simulink model "qpsk"  (R2021a)
settings: Solver=FixedStepDiscrete  StartTime=0.0  StopTime=1e-3  FixedStep=1/sampling_freq  RelTol=1e-3
undefined symbols (not defined in the file): coeff, data_rate, nco_21, sample_ratio, sampling_freq
libraries: simulink x6, simulink_extras x5, dspswit3 x2, commchan3 x1, commrandsrc2 x1, commsink2 x1
settings Model: SimulationMode=accelerator  Creator=Administrator  LastModifiedBy=Administrator

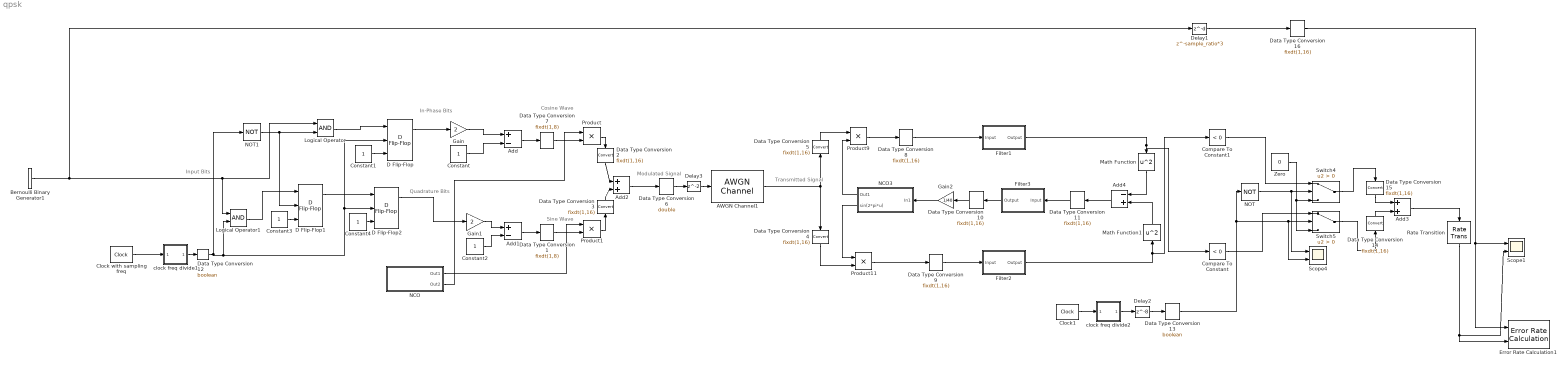
== system qpsk ==
  note: Transmitted Signal
  note: Quadrature Bits
  note: In-Phase Bits
  note: Input Bits
  note: Modulated Signal
  note: Cosine Wave
  note: Sine Wave
  AWGN Channel1 : commchan3/AWGN Channel  InputProcessing=Columns as channels (frame based)  seed=532  noiseMode="Signal to noise ratio  (Eb/No)"  EbNodB=SNR  EsNodB=10  SNRdB=SNR  bitsPerSym=1  Ps=1  Tsym=1/data_rate  variance=1
  Add : Sum  Inputs=+-
  Add1 : Sum  Inputs=+-
  Add2 : Sum
  Add3 : Sum
  Add4 : Sum  Inputs=-+
  Bernoulli Binary Generator1 : commrandsrc2/Bernoulli Binary Generator  P=0.3  seed=14  Ts=1/data_rate  frameBased=off  sampPerFrame=1  orient=off  outDataType=boolean
      settings: SourceProductBaseCode=CM
  Clock with sampling freq : simulink_extras/Flip Flops/Clock  period=1/sampling_freq*2
  Clock1 : simulink_extras/Flip Flops/Clock  period=1/sampling_freq*2
  Compare To Constant : simulink/Logic and Bit Operations/Compare To Constant  relop=<  const=0  OutDataTypeStr=boolean
  Compare To Constant1 : simulink/Logic and Bit Operations/Compare To Constant  relop=<  const=0  OutDataTypeStr=boolean
  Constant : Constant
  Constant1 : Constant  OutDataTypeStr=boolean
  Constant2 : Constant
  Constant3 : Constant  OutDataTypeStr=boolean
  Constant4 : Constant  OutDataTypeStr=boolean
  D Flip-Flop : simulink_extras/Flip Flops/D Flip-Flop
  D Flip-Flop1 : simulink_extras/Flip Flops/D Flip-Flop
  D Flip-Flop2 : simulink_extras/Flip Flops/D Flip-Flop
  Data Type Conversion1 : DataTypeConversion  OutMax=[1]  OutDataTypeStr=fixdt(1,8)
  Data Type Conversion{2..5,8..11,14..16} (11 alike) : DataTypeConversion  OutMax=[1]  OutDataTypeStr=fixdt(1,16)
  Data Type Conversion12 : DataTypeConversion  OutMax=[1]  OutDataTypeStr=boolean
  Data Type Conversion13 : DataTypeConversion  OutMax=[1]  OutDataTypeStr=boolean
  Data Type Conversion6 : DataTypeConversion  OutDataTypeStr=double  LockScale=on
  Data Type Conversion7 : DataTypeConversion  OutMax=[1]  OutDataTypeStr=fixdt(1,8)
  Delay1 : Delay  DelayLength=sample_ratio*3  SampleTime=1/sampling_freq
  Delay2 : Delay  DelayLength=8  SampleTime=1/sampling_freq
  Delay3 : Delay  SampleTime=1/sampling_freq
  Error Rate Calculation1 : commsink2/Error Rate Calculation  N=0  st_delay=20000  cp_mode=Entire frame  subframe=[]  PMode=Workspace  WsName=ErrorVec_QPSK  RsMode2=off  stop=off  numErr=100  maxBits=1e6
  Filter1 : Subsystem  Tag=FilterWizardSubSystem
      settings: ErrorFcn=dspFilterRealizedInBasicElemsAlgLoopErrFcnCallback
  Filter2 : Subsystem  Tag=FilterWizardSubSystem
      settings: ErrorFcn=dspFilterRealizedInBasicElemsAlgLoopErrFcnCallback
  Filter3 : Subsystem  Tag=FilterWizardSubSystem
      settings: ErrorFcn=dspFilterRealizedInBasicElemsAlgLoopErrFcnCallback
  Gain : Gain  Gain=2
  Gain1 : Gain  Gain=2
  Gain2 : Gain  Gain=1/40
  Logical Operator : Logic  AllPortsSameDT=off  OutDataTypeStr=boolean
  Logical Operator1 : Logic  AllPortsSameDT=off  OutDataTypeStr=boolean
  Math Function : Math  Operator=square  SignedPower=on  SaturateOnIntegerOverflow=on
  Math Function1 : Math  Operator=square  SignedPower=on  SaturateOnIntegerOverflow=on
  NCO : Subsystem
  NCO3 : Subsystem
  NOT : Logic  Operator=NOT  IconShape=distinctive  AllPortsSameDT=off  OutDataTypeStr=boolean
  NOT1 : Logic  Operator=NOT  IconShape=distinctive  AllPortsSameDT=off  OutDataTypeStr=boolean
  Product{,1,9,11} (4 alike) : Product
  Rate Transition : RateTransition  OutPortSampleTime=1/data_rate
  Scope1 : Scope  NumInputPorts=2
  Scope4 : Scope  NumInputPorts=2
  Switch4 : Switch  Criteria=u2 > Threshold
  Switch5 : Switch  Criteria=u2 > Threshold
  Zero : Constant  Value=0  OutDataTypeStr=fixdt(1,16,12)
  clock freq divide1 : Subsystem
  clock freq divide2 : Subsystem
  wires:
  Constant/1 -> Add/2
  Gain/1 -> Add/1
  Gain1/1 -> Add1/1
  Constant2/1 -> Add1/2
  Add/1 -> Data Type Conversion7/1
  Add1/1 -> Data Type Conversion1/1
  Product/1 -> Data Type Conversion2/1
  Product1/1 -> Data Type Conversion3/1
  Add2/1 -> Data Type Conversion6/1
  Product9/1 -> Data Type Conversion8/1
  Product11/1 -> Data Type Conversion9/1
  AWGN Channel1/1 -> Data Type Conversion4/1, Data Type Conversion5/1
  Data Type Conversion7/1 -> Product/2
  Data Type Conversion1/1 -> Product1/2
  Data Type Conversion2/1 -> Add2/1
  Data Type Conversion3/1 -> Add2/2
  Data Type Conversion4/1 -> Product11/2
  Data Type Conversion5/1 -> Product9/1
  Data Type Conversion6/1 -> Delay3/1
  NCO3/1(Out1) -> Product9/2
  NCO3/2(sin(2*pi*u)) -> Product11/1
  NCO/2(Out2) -> Product/1
  Data Type Conversion8/1 -> Filter1/1(Input)
  Data Type Conversion9/1 -> Filter2/1(Input)
  Gain2/1 -> NCO3/1(In1)
  Data Type Conversion11/1 -> Filter3/1(Input)
  Constant4/1 -> D Flip-Flop2/3
  D Flip-Flop/1 -> Gain/1
  Constant1/1 -> D Flip-Flop/3
  Constant3/1 -> D Flip-Flop1/3
  Logical Operator/1 -> D Flip-Flop/1
  NOT1/1 -> D Flip-Flop1/2, Logical Operator/2
  Logical Operator1/1 -> D Flip-Flop1/1
  D Flip-Flop2/1 -> Gain1/1
  D Flip-Flop1/1 -> D Flip-Flop2/1
  Clock with sampling freq/1 -> clock freq divide1/1(In1)
  Data Type Conversion12/1 -> NOT1/1, D Flip-Flop/2, D Flip-Flop2/2, Logical Operator1/2
  Delay1/1 -> Data Type Conversion16/1
  Delay2/1 -> Data Type Conversion13/1
  Compare To Constant1/1 -> Switch4/1
  Data Type Conversion14/1 -> Add3/2
  Data Type Conversion15/1 -> Add3/1
  Data Type Conversion16/1 -> Error Rate Calculation1/1, Scope1/1
  Add3/1 -> Rate Transition/1
  NCO/1(Out1) -> Product1/1
  Math Function/1 -> Add4/1
  Math Function1/1 -> Add4/2
  Add4/1 -> Data Type Conversion11/1
  Data Type Conversion13/1 -> NOT/1, Scope4/2, Switch5/2
  NOT/1 -> Scope4/1, Switch4/2
  Compare To Constant/1 -> Switch5/1
  Zero/1 -> Switch5/3, Switch4/3
  Switch4/1 -> Data Type Conversion15/1
  Switch5/1 -> Data Type Conversion14/1
  Delay3/1 -> AWGN Channel1/1
  Filter1/1(Output) -> Compare To Constant/1, Math Function/1
  Filter2/1(Output) -> Compare To Constant1/1, Math Function1/1
  Filter3/1(Output) -> Data Type Conversion10/1
  Data Type Conversion10/1 -> Gain2/1
  Bernoulli Binary Generator1/1 -> Logical Operator/1, Logical Operator1/1, Delay1/1
  Rate Transition/1 -> Scope1/2, Error Rate Calculation1/2
  clock freq divide1/1(Out1) -> Data Type Conversion12/1
  Clock1/1 -> clock freq divide2/1(In1)
  clock freq divide2/1(Out1) -> Delay2/1

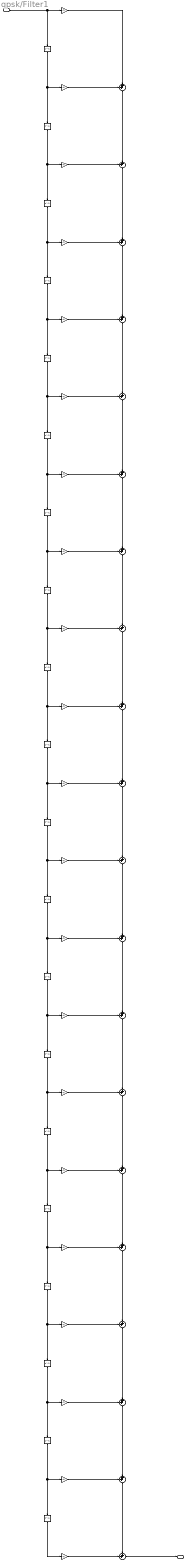
== system qpsk/Filter1 ==
  Input : Inport
  BodyDelay{2..21} (20 alike) : Delay  DelayLength=1  InitialCondition=0  InputProcessing=Columns as channels (frame based)  SampleTime=1/sampling_freq
  BodyLSum{2..21} (20 alike) : Sum  Inputs=++|  RndMeth=Nearest  SaturateOnIntegerOverflow=on  OutDataTypeStr=Inherit: Same as first input
  b(1) : Gain  Gain=coeff(1)  ParamDataTypeStr=double  RndMeth=Nearest  SaturateOnIntegerOverflow=on  OutDataTypeStr=Inherit: Same as input
  b(10) : Gain  Gain=coeff(10)  ParamDataTypeStr=double  RndMeth=Nearest  SaturateOnIntegerOverflow=on  OutDataTypeStr=Inherit: Same as input
  b(11) : Gain  Gain=coeff(11)  ParamDataTypeStr=double  RndMeth=Nearest  SaturateOnIntegerOverflow=on  OutDataTypeStr=Inherit: Same as input
  b(12) : Gain  Gain=coeff(12)  ParamDataTypeStr=double  RndMeth=Nearest  SaturateOnIntegerOverflow=on  OutDataTypeStr=Inherit: Same as input
  b(13) : Gain  Gain=coeff(13)  ParamDataTypeStr=double  RndMeth=Nearest  SaturateOnIntegerOverflow=on  OutDataTypeStr=Inherit: Same as input
  b(14) : Gain  Gain=coeff(14)  ParamDataTypeStr=double  RndMeth=Nearest  SaturateOnIntegerOverflow=on  OutDataTypeStr=Inherit: Same as input
  b(15) : Gain  Gain=coeff(15)  ParamDataTypeStr=double  RndMeth=Nearest  SaturateOnIntegerOverflow=on  OutDataTypeStr=Inherit: Same as input
  b(16) : Gain  Gain=coeff(16)  ParamDataTypeStr=double  RndMeth=Nearest  SaturateOnIntegerOverflow=on  OutDataTypeStr=Inherit: Same as input
  b(17) : Gain  Gain=coeff(17)  ParamDataTypeStr=double  RndMeth=Nearest  SaturateOnIntegerOverflow=on  OutDataTypeStr=Inherit: Same as input
  b(18) : Gain  Gain=coeff(18)  ParamDataTypeStr=double  RndMeth=Nearest  SaturateOnIntegerOverflow=on  OutDataTypeStr=Inherit: Same as input
  b(19) : Gain  Gain=coeff(19)  ParamDataTypeStr=double  RndMeth=Nearest  SaturateOnIntegerOverflow=on  OutDataTypeStr=Inherit: Same as input
  b(2) : Gain  Gain=coeff(2)  ParamDataTypeStr=double  RndMeth=Nearest  SaturateOnIntegerOverflow=on  OutDataTypeStr=Inherit: Same as input
  b(20) : Gain  Gain=coeff(20)  ParamDataTypeStr=double  RndMeth=Nearest  SaturateOnIntegerOverflow=on  OutDataTypeStr=Inherit: Same as input
  b(21) : Gain  Gain=coeff(21)  ParamDataTypeStr=double  RndMeth=Nearest  SaturateOnIntegerOverflow=on  OutDataTypeStr=Inherit: Same as input
  b(3) : Gain  Gain=coeff(3)  ParamDataTypeStr=double  RndMeth=Nearest  SaturateOnIntegerOverflow=on  OutDataTypeStr=Inherit: Same as input
  b(4) : Gain  Gain=coeff(4)  ParamDataTypeStr=double  RndMeth=Nearest  SaturateOnIntegerOverflow=on  OutDataTypeStr=Inherit: Same as input
  b(5) : Gain  Gain=coeff(5)  ParamDataTypeStr=double  RndMeth=Nearest  SaturateOnIntegerOverflow=on  OutDataTypeStr=Inherit: Same as input
  b(6) : Gain  Gain=coeff(6)  ParamDataTypeStr=double  RndMeth=Nearest  SaturateOnIntegerOverflow=on  OutDataTypeStr=Inherit: Same as input
  b(7) : Gain  Gain=coeff(7)  ParamDataTypeStr=double  RndMeth=Nearest  SaturateOnIntegerOverflow=on  OutDataTypeStr=Inherit: Same as input
  b(8) : Gain  Gain=coeff(8)  ParamDataTypeStr=double  RndMeth=Nearest  SaturateOnIntegerOverflow=on  OutDataTypeStr=Inherit: Same as input
  b(9) : Gain  Gain=coeff(9)  ParamDataTypeStr=double  RndMeth=Nearest  SaturateOnIntegerOverflow=on  OutDataTypeStr=Inherit: Same as input
  Output : Outport
  wires:
  Input/1 -> b(1)/1, BodyDelay2/1
  b(1)/1 -> BodyLSum2/2
  BodyDelay2/1 -> b(2)/1, BodyDelay3/1
  b(2)/1 -> BodyLSum2/1
  BodyLSum2/1 -> BodyLSum3/2
  BodyDelay3/1 -> b(3)/1, BodyDelay4/1
  b(3)/1 -> BodyLSum3/1
  BodyLSum3/1 -> BodyLSum4/2
  BodyDelay4/1 -> b(4)/1, BodyDelay5/1
  b(4)/1 -> BodyLSum4/1
  BodyLSum4/1 -> BodyLSum5/2
  BodyDelay5/1 -> b(5)/1, BodyDelay6/1
  b(5)/1 -> BodyLSum5/1
  BodyLSum5/1 -> BodyLSum6/2
  BodyDelay6/1 -> b(6)/1, BodyDelay7/1
  b(6)/1 -> BodyLSum6/1
  BodyLSum6/1 -> BodyLSum7/2
  BodyDelay7/1 -> b(7)/1, BodyDelay8/1
  b(7)/1 -> BodyLSum7/1
  BodyLSum7/1 -> BodyLSum8/2
  BodyDelay8/1 -> b(8)/1, BodyDelay9/1
  b(8)/1 -> BodyLSum8/1
  BodyLSum8/1 -> BodyLSum9/2
  BodyDelay9/1 -> b(9)/1, BodyDelay10/1
  b(9)/1 -> BodyLSum9/1
  BodyLSum9/1 -> BodyLSum10/2
  BodyDelay10/1 -> b(10)/1, BodyDelay11/1
  b(10)/1 -> BodyLSum10/1
  BodyLSum10/1 -> BodyLSum11/2
  BodyDelay11/1 -> b(11)/1, BodyDelay12/1
  b(11)/1 -> BodyLSum11/1
  BodyLSum11/1 -> BodyLSum12/2
  BodyDelay12/1 -> b(12)/1, BodyDelay13/1
  b(12)/1 -> BodyLSum12/1
  BodyLSum12/1 -> BodyLSum13/2
  BodyDelay13/1 -> b(13)/1, BodyDelay14/1
  b(13)/1 -> BodyLSum13/1
  BodyLSum13/1 -> BodyLSum14/2
  BodyDelay14/1 -> b(14)/1, BodyDelay15/1
  b(14)/1 -> BodyLSum14/1
  BodyLSum14/1 -> BodyLSum15/2
  BodyDelay15/1 -> b(15)/1, BodyDelay16/1
  b(15)/1 -> BodyLSum15/1
  BodyLSum15/1 -> BodyLSum16/2
  BodyDelay16/1 -> b(16)/1, BodyDelay17/1
  b(16)/1 -> BodyLSum16/1
  BodyLSum16/1 -> BodyLSum17/2
  BodyDelay17/1 -> b(17)/1, BodyDelay18/1
  b(17)/1 -> BodyLSum17/1
  BodyLSum17/1 -> BodyLSum18/2
  BodyDelay18/1 -> b(18)/1, BodyDelay19/1
  b(18)/1 -> BodyLSum18/1
  BodyLSum18/1 -> BodyLSum19/2
  BodyDelay19/1 -> b(19)/1, BodyDelay20/1
  b(19)/1 -> BodyLSum19/1
  BodyLSum19/1 -> BodyLSum20/2
  BodyDelay20/1 -> b(20)/1, BodyDelay21/1
  b(20)/1 -> BodyLSum20/1
  BodyLSum20/1 -> BodyLSum21/1
  BodyDelay21/1 -> b(21)/1
  b(21)/1 -> BodyLSum21/2
  BodyLSum21/1 -> Output/1

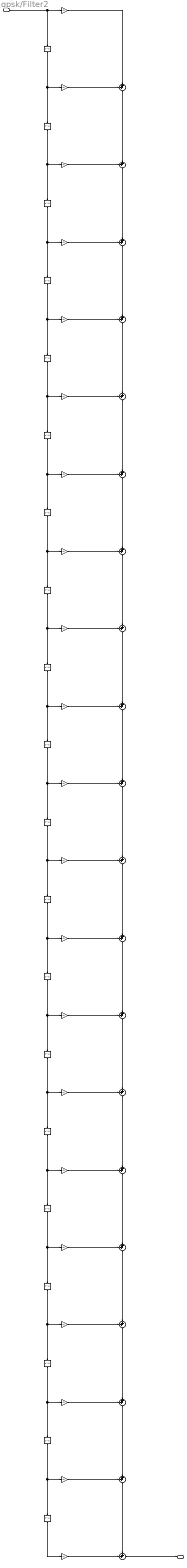
== system qpsk/Filter2 ==
  Input : Inport
  BodyDelay{2..21} (20 alike) : Delay  DelayLength=1  InitialCondition=0  InputProcessing=Columns as channels (frame based)  SampleTime=1/sampling_freq
  BodyLSum{2..21} (20 alike) : Sum  Inputs=++|  RndMeth=Nearest  SaturateOnIntegerOverflow=on  OutDataTypeStr=Inherit: Same as first input
  b(1) : Gain  Gain=coeff(1)  ParamDataTypeStr=double  RndMeth=Nearest  SaturateOnIntegerOverflow=on  OutDataTypeStr=Inherit: Same as input
  b(10) : Gain  Gain=coeff(10)  ParamDataTypeStr=double  RndMeth=Nearest  SaturateOnIntegerOverflow=on  OutDataTypeStr=Inherit: Same as input
  b(11) : Gain  Gain=coeff(11)  ParamDataTypeStr=double  RndMeth=Nearest  SaturateOnIntegerOverflow=on  OutDataTypeStr=Inherit: Same as input
  b(12) : Gain  Gain=coeff(12)  ParamDataTypeStr=double  RndMeth=Nearest  SaturateOnIntegerOverflow=on  OutDataTypeStr=Inherit: Same as input
  b(13) : Gain  Gain=coeff(13)  ParamDataTypeStr=double  RndMeth=Nearest  SaturateOnIntegerOverflow=on  OutDataTypeStr=Inherit: Same as input
  b(14) : Gain  Gain=coeff(14)  ParamDataTypeStr=double  RndMeth=Nearest  SaturateOnIntegerOverflow=on  OutDataTypeStr=Inherit: Same as input
  b(15) : Gain  Gain=coeff(15)  ParamDataTypeStr=double  RndMeth=Nearest  SaturateOnIntegerOverflow=on  OutDataTypeStr=Inherit: Same as input
  b(16) : Gain  Gain=coeff(16)  ParamDataTypeStr=double  RndMeth=Nearest  SaturateOnIntegerOverflow=on  OutDataTypeStr=Inherit: Same as input
  b(17) : Gain  Gain=coeff(17)  ParamDataTypeStr=double  RndMeth=Nearest  SaturateOnIntegerOverflow=on  OutDataTypeStr=Inherit: Same as input
  b(18) : Gain  Gain=coeff(18)  ParamDataTypeStr=double  RndMeth=Nearest  SaturateOnIntegerOverflow=on  OutDataTypeStr=Inherit: Same as input
  b(19) : Gain  Gain=coeff(19)  ParamDataTypeStr=double  RndMeth=Nearest  SaturateOnIntegerOverflow=on  OutDataTypeStr=Inherit: Same as input
  b(2) : Gain  Gain=coeff(2)  ParamDataTypeStr=double  RndMeth=Nearest  SaturateOnIntegerOverflow=on  OutDataTypeStr=Inherit: Same as input
  b(20) : Gain  Gain=coeff(20)  ParamDataTypeStr=double  RndMeth=Nearest  SaturateOnIntegerOverflow=on  OutDataTypeStr=Inherit: Same as input
  b(21) : Gain  Gain=coeff(21)  ParamDataTypeStr=double  RndMeth=Nearest  SaturateOnIntegerOverflow=on  OutDataTypeStr=Inherit: Same as input
  b(3) : Gain  Gain=coeff(3)  ParamDataTypeStr=double  RndMeth=Nearest  SaturateOnIntegerOverflow=on  OutDataTypeStr=Inherit: Same as input
  b(4) : Gain  Gain=coeff(4)  ParamDataTypeStr=double  RndMeth=Nearest  SaturateOnIntegerOverflow=on  OutDataTypeStr=Inherit: Same as input
  b(5) : Gain  Gain=coeff(5)  ParamDataTypeStr=double  RndMeth=Nearest  SaturateOnIntegerOverflow=on  OutDataTypeStr=Inherit: Same as input
  b(6) : Gain  Gain=coeff(6)  ParamDataTypeStr=double  RndMeth=Nearest  SaturateOnIntegerOverflow=on  OutDataTypeStr=Inherit: Same as input
  b(7) : Gain  Gain=coeff(7)  ParamDataTypeStr=double  RndMeth=Nearest  SaturateOnIntegerOverflow=on  OutDataTypeStr=Inherit: Same as input
  b(8) : Gain  Gain=coeff(8)  ParamDataTypeStr=double  RndMeth=Nearest  SaturateOnIntegerOverflow=on  OutDataTypeStr=Inherit: Same as input
  b(9) : Gain  Gain=coeff(9)  ParamDataTypeStr=double  RndMeth=Nearest  SaturateOnIntegerOverflow=on  OutDataTypeStr=Inherit: Same as input
  Output : Outport
  wires:
  Input/1 -> b(1)/1, BodyDelay2/1
  b(1)/1 -> BodyLSum2/2
  BodyDelay2/1 -> b(2)/1, BodyDelay3/1
  b(2)/1 -> BodyLSum2/1
  BodyLSum2/1 -> BodyLSum3/2
  BodyDelay3/1 -> b(3)/1, BodyDelay4/1
  b(3)/1 -> BodyLSum3/1
  BodyLSum3/1 -> BodyLSum4/2
  BodyDelay4/1 -> b(4)/1, BodyDelay5/1
  b(4)/1 -> BodyLSum4/1
  BodyLSum4/1 -> BodyLSum5/2
  BodyDelay5/1 -> b(5)/1, BodyDelay6/1
  b(5)/1 -> BodyLSum5/1
  BodyLSum5/1 -> BodyLSum6/2
  BodyDelay6/1 -> b(6)/1, BodyDelay7/1
  b(6)/1 -> BodyLSum6/1
  BodyLSum6/1 -> BodyLSum7/2
  BodyDelay7/1 -> b(7)/1, BodyDelay8/1
  b(7)/1 -> BodyLSum7/1
  BodyLSum7/1 -> BodyLSum8/2
  BodyDelay8/1 -> b(8)/1, BodyDelay9/1
  b(8)/1 -> BodyLSum8/1
  BodyLSum8/1 -> BodyLSum9/2
  BodyDelay9/1 -> b(9)/1, BodyDelay10/1
  b(9)/1 -> BodyLSum9/1
  BodyLSum9/1 -> BodyLSum10/2
  BodyDelay10/1 -> b(10)/1, BodyDelay11/1
  b(10)/1 -> BodyLSum10/1
  BodyLSum10/1 -> BodyLSum11/2
  BodyDelay11/1 -> b(11)/1, BodyDelay12/1
  b(11)/1 -> BodyLSum11/1
  BodyLSum11/1 -> BodyLSum12/2
  BodyDelay12/1 -> b(12)/1, BodyDelay13/1
  b(12)/1 -> BodyLSum12/1
  BodyLSum12/1 -> BodyLSum13/2
  BodyDelay13/1 -> b(13)/1, BodyDelay14/1
  b(13)/1 -> BodyLSum13/1
  BodyLSum13/1 -> BodyLSum14/2
  BodyDelay14/1 -> b(14)/1, BodyDelay15/1
  b(14)/1 -> BodyLSum14/1
  BodyLSum14/1 -> BodyLSum15/2
  BodyDelay15/1 -> b(15)/1, BodyDelay16/1
  b(15)/1 -> BodyLSum15/1
  BodyLSum15/1 -> BodyLSum16/2
  BodyDelay16/1 -> b(16)/1, BodyDelay17/1
  b(16)/1 -> BodyLSum16/1
  BodyLSum16/1 -> BodyLSum17/2
  BodyDelay17/1 -> b(17)/1, BodyDelay18/1
  b(17)/1 -> BodyLSum17/1
  BodyLSum17/1 -> BodyLSum18/2
  BodyDelay18/1 -> b(18)/1, BodyDelay19/1
  b(18)/1 -> BodyLSum18/1
  BodyLSum18/1 -> BodyLSum19/2
  BodyDelay19/1 -> b(19)/1, BodyDelay20/1
  b(19)/1 -> BodyLSum19/1
  BodyLSum19/1 -> BodyLSum20/2
  BodyDelay20/1 -> b(20)/1, BodyDelay21/1
  b(20)/1 -> BodyLSum20/1
  BodyLSum20/1 -> BodyLSum21/1
  BodyDelay21/1 -> b(21)/1
  b(21)/1 -> BodyLSum21/2
  BodyLSum21/1 -> Output/1

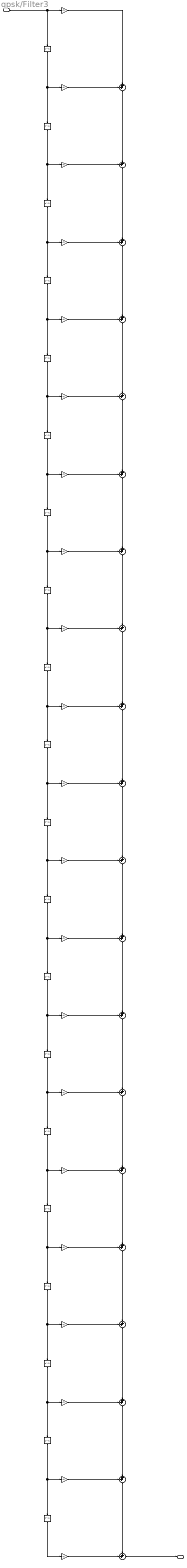
== system qpsk/Filter3 ==
  Input : Inport
  BodyDelay{2..21} (20 alike) : Delay  DelayLength=1  InitialCondition=0  InputProcessing=Columns as channels (frame based)  SampleTime=1/sampling_freq
  BodyLSum{2..21} (20 alike) : Sum  Inputs=++|  RndMeth=Nearest  SaturateOnIntegerOverflow=on  OutDataTypeStr=Inherit: Same as first input
  b(1) : Gain  Gain=coeff(1)  ParamDataTypeStr=double  RndMeth=Nearest  SaturateOnIntegerOverflow=on  OutDataTypeStr=Inherit: Same as input
  b(10) : Gain  Gain=coeff(10)  ParamDataTypeStr=double  RndMeth=Nearest  SaturateOnIntegerOverflow=on  OutDataTypeStr=Inherit: Same as input
  b(11) : Gain  Gain=coeff(11)  ParamDataTypeStr=double  RndMeth=Nearest  SaturateOnIntegerOverflow=on  OutDataTypeStr=Inherit: Same as input
  b(12) : Gain  Gain=coeff(12)  ParamDataTypeStr=double  RndMeth=Nearest  SaturateOnIntegerOverflow=on  OutDataTypeStr=Inherit: Same as input
  b(13) : Gain  Gain=coeff(13)  ParamDataTypeStr=double  RndMeth=Nearest  SaturateOnIntegerOverflow=on  OutDataTypeStr=Inherit: Same as input
  b(14) : Gain  Gain=coeff(14)  ParamDataTypeStr=double  RndMeth=Nearest  SaturateOnIntegerOverflow=on  OutDataTypeStr=Inherit: Same as input
  b(15) : Gain  Gain=coeff(15)  ParamDataTypeStr=double  RndMeth=Nearest  SaturateOnIntegerOverflow=on  OutDataTypeStr=Inherit: Same as input
  b(16) : Gain  Gain=coeff(16)  ParamDataTypeStr=double  RndMeth=Nearest  SaturateOnIntegerOverflow=on  OutDataTypeStr=Inherit: Same as input
  b(17) : Gain  Gain=coeff(17)  ParamDataTypeStr=double  RndMeth=Nearest  SaturateOnIntegerOverflow=on  OutDataTypeStr=Inherit: Same as input
  b(18) : Gain  Gain=coeff(18)  ParamDataTypeStr=double  RndMeth=Nearest  SaturateOnIntegerOverflow=on  OutDataTypeStr=Inherit: Same as input
  b(19) : Gain  Gain=coeff(19)  ParamDataTypeStr=double  RndMeth=Nearest  SaturateOnIntegerOverflow=on  OutDataTypeStr=Inherit: Same as input
  b(2) : Gain  Gain=coeff(2)  ParamDataTypeStr=double  RndMeth=Nearest  SaturateOnIntegerOverflow=on  OutDataTypeStr=Inherit: Same as input
  b(20) : Gain  Gain=coeff(20)  ParamDataTypeStr=double  RndMeth=Nearest  SaturateOnIntegerOverflow=on  OutDataTypeStr=Inherit: Same as input
  b(21) : Gain  Gain=coeff(21)  ParamDataTypeStr=double  RndMeth=Nearest  SaturateOnIntegerOverflow=on  OutDataTypeStr=Inherit: Same as input
  b(3) : Gain  Gain=coeff(3)  ParamDataTypeStr=double  RndMeth=Nearest  SaturateOnIntegerOverflow=on  OutDataTypeStr=Inherit: Same as input
  b(4) : Gain  Gain=coeff(4)  ParamDataTypeStr=double  RndMeth=Nearest  SaturateOnIntegerOverflow=on  OutDataTypeStr=Inherit: Same as input
  b(5) : Gain  Gain=coeff(5)  ParamDataTypeStr=double  RndMeth=Nearest  SaturateOnIntegerOverflow=on  OutDataTypeStr=Inherit: Same as input
  b(6) : Gain  Gain=coeff(6)  ParamDataTypeStr=double  RndMeth=Nearest  SaturateOnIntegerOverflow=on  OutDataTypeStr=Inherit: Same as input
  b(7) : Gain  Gain=coeff(7)  ParamDataTypeStr=double  RndMeth=Nearest  SaturateOnIntegerOverflow=on  OutDataTypeStr=Inherit: Same as input
  b(8) : Gain  Gain=coeff(8)  ParamDataTypeStr=double  RndMeth=Nearest  SaturateOnIntegerOverflow=on  OutDataTypeStr=Inherit: Same as input
  b(9) : Gain  Gain=coeff(9)  ParamDataTypeStr=double  RndMeth=Nearest  SaturateOnIntegerOverflow=on  OutDataTypeStr=Inherit: Same as input
  Output : Outport
  wires:
  Input/1 -> b(1)/1, BodyDelay2/1
  b(1)/1 -> BodyLSum2/2
  BodyDelay2/1 -> b(2)/1, BodyDelay3/1
  b(2)/1 -> BodyLSum2/1
  BodyLSum2/1 -> BodyLSum3/2
  BodyDelay3/1 -> b(3)/1, BodyDelay4/1
  b(3)/1 -> BodyLSum3/1
  BodyLSum3/1 -> BodyLSum4/2
  BodyDelay4/1 -> b(4)/1, BodyDelay5/1
  b(4)/1 -> BodyLSum4/1
  BodyLSum4/1 -> BodyLSum5/2
  BodyDelay5/1 -> b(5)/1, BodyDelay6/1
  b(5)/1 -> BodyLSum5/1
  BodyLSum5/1 -> BodyLSum6/2
  BodyDelay6/1 -> b(6)/1, BodyDelay7/1
  b(6)/1 -> BodyLSum6/1
  BodyLSum6/1 -> BodyLSum7/2
  BodyDelay7/1 -> b(7)/1, BodyDelay8/1
  b(7)/1 -> BodyLSum7/1
  BodyLSum7/1 -> BodyLSum8/2
  BodyDelay8/1 -> b(8)/1, BodyDelay9/1
  b(8)/1 -> BodyLSum8/1
  BodyLSum8/1 -> BodyLSum9/2
  BodyDelay9/1 -> b(9)/1, BodyDelay10/1
  b(9)/1 -> BodyLSum9/1
  BodyLSum9/1 -> BodyLSum10/2
  BodyDelay10/1 -> b(10)/1, BodyDelay11/1
  b(10)/1 -> BodyLSum10/1
  BodyLSum10/1 -> BodyLSum11/2
  BodyDelay11/1 -> b(11)/1, BodyDelay12/1
  b(11)/1 -> BodyLSum11/1
  BodyLSum11/1 -> BodyLSum12/2
  BodyDelay12/1 -> b(12)/1, BodyDelay13/1
  b(12)/1 -> BodyLSum12/1
  BodyLSum12/1 -> BodyLSum13/2
  BodyDelay13/1 -> b(13)/1, BodyDelay14/1
  b(13)/1 -> BodyLSum13/1
  BodyLSum13/1 -> BodyLSum14/2
  BodyDelay14/1 -> b(14)/1, BodyDelay15/1
  b(14)/1 -> BodyLSum14/1
  BodyLSum14/1 -> BodyLSum15/2
  BodyDelay15/1 -> b(15)/1, BodyDelay16/1
  b(15)/1 -> BodyLSum15/1
  BodyLSum15/1 -> BodyLSum16/2
  BodyDelay16/1 -> b(16)/1, BodyDelay17/1
  b(16)/1 -> BodyLSum16/1
  BodyLSum16/1 -> BodyLSum17/2
  BodyDelay17/1 -> b(17)/1, BodyDelay18/1
  b(17)/1 -> BodyLSum17/1
  BodyLSum17/1 -> BodyLSum18/2
  BodyDelay18/1 -> b(18)/1, BodyDelay19/1
  b(18)/1 -> BodyLSum18/1
  BodyLSum18/1 -> BodyLSum19/2
  BodyDelay19/1 -> b(19)/1, BodyDelay20/1
  b(19)/1 -> BodyLSum19/1
  BodyLSum19/1 -> BodyLSum20/2
  BodyDelay20/1 -> b(20)/1, BodyDelay21/1
  b(20)/1 -> BodyLSum20/1
  BodyLSum20/1 -> BodyLSum21/1
  BodyDelay21/1 -> b(21)/1
  b(21)/1 -> BodyLSum21/2
  BodyLSum21/1 -> Output/1

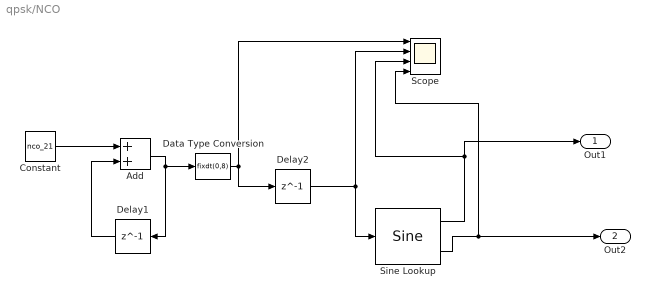
== system qpsk/NCO ==
  Add : Sum  AccumDataTypeStr=double
  Constant : Constant  Value=nco_21  OutDataTypeStr=double  SampleTime=1/sampling_freq
  Data Type Conversion : DataTypeConversion  OutMin=[0]  OutMax=[2]  OutDataTypeStr=fixdt(0,8)
  Delay1 : Delay  DelayLength=1  InitialCondition=0  UseCircularBuffer=on  SampleTime=1/sampling_freq
  Delay2 : Delay  DelayLength=1  InitialCondition=0  UseCircularBuffer=on  SampleTime=1/sampling_freq
  Scope : Scope  NumInputPorts=4
  Sine Lookup : simulink/Lookup Tables/Sine  Formula=sin(2*pi*u) and cos(2*pi*u)  NumDataPoints=(2^3)+1  OutputWordLength=8  InternalRulePriority=Speed
  Out1 : Outport
  Out2 : Outport  Port=2
  wires:
  Delay1/1 -> Add/2
  Constant/1 -> Add/1
  Add/1 -> Delay1/1, Data Type Conversion/1
  Sine Lookup/1 -> Out1/1, Scope/3
  Sine Lookup/2 -> Out2/1, Scope/4
  Data Type Conversion/1 -> Delay2/1, Scope/1
  Delay2/1 -> Scope/2, Sine Lookup/1

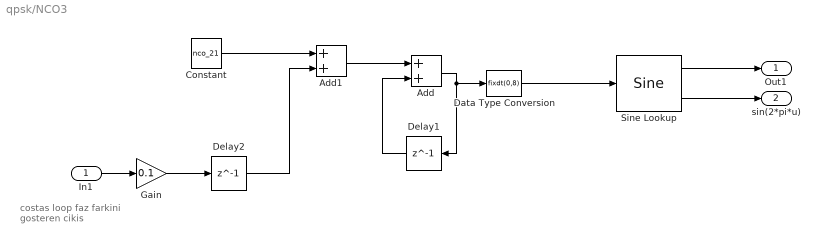
== system qpsk/NCO3 ==
  note: costas loop faz farkini gosteren cikis
  In1 : Inport
  Add : Sum  AccumDataTypeStr=double
  Add1 : Sum
  Constant : Constant  Value=nco_21  OutDataTypeStr=double  SampleTime=1/sampling_freq
  Data Type Conversion : DataTypeConversion  OutMin=[0]  OutMax=[2]  OutDataTypeStr=fixdt(0,8)
  Delay1 : Delay  DelayLength=1  InitialCondition=0  UseCircularBuffer=on  SampleTime=1/sampling_freq
  Delay2 : Delay  DelayLength=1  InitialCondition=0  UseCircularBuffer=on  SampleTime=1/sampling_freq
  Gain : Gain  Gain=0.1
  Sine Lookup : simulink/Lookup Tables/Sine  Formula=sin(2*pi*u) and cos(2*pi*u)  NumDataPoints=(2^3)+1  OutputWordLength=8  InternalRulePriority=Speed
  Out1 : Outport
  sin(2*pi*u) : Outport  Port=2
  wires:
  Sine Lookup/2 -> sin(2*pi*u)/1
  Sine Lookup/1 -> Out1/1
  Delay1/1 -> Add/2
  Add/1 -> Delay1/1, Data Type Conversion/1
  Add1/1 -> Add/1
  Constant/1 -> Add1/1
  Gain/1 -> Delay2/1
  In1/1 -> Gain/1
  Data Type Conversion/1 -> Sine Lookup/1
  Delay2/1 -> Add1/2

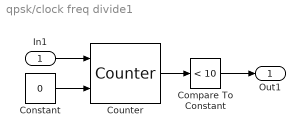
== system qpsk/clock freq divide1 ==
  In1 : Inport
  Compare To Constant : simulink/Logic and Bit Operations/Compare To Constant  relop=<  const=10  OutDataTypeStr=boolean
  Constant : Constant  Value=0
  Counter : dspswit3/Counter  Direction=Up  CountEvent=Rising edge  CounterSize=User defined  MaxCount=19  InitialCount=0  Output=Count  HitValue=19  ResetInput=on  SamplesPerFrame=1  Ts=1  CntDtype=int8  HitDtype=Logical
  Out1 : Outport
  wires:
  Counter/1 -> Compare To Constant/1
  Constant/1 -> Counter/2
  Compare To Constant/1 -> Out1/1
  In1/1 -> Counter/1

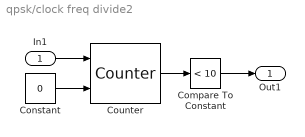
== system qpsk/clock freq divide2 ==
  In1 : Inport
  Compare To Constant : simulink/Logic and Bit Operations/Compare To Constant  relop=<  const=10  OutDataTypeStr=boolean
  Constant : Constant  Value=0
  Counter : dspswit3/Counter  Direction=Up  CountEvent=Rising edge  CounterSize=User defined  MaxCount=19  InitialCount=0  Output=Count  HitValue=19  ResetInput=on  SamplesPerFrame=1  Ts=1  CntDtype=int8  HitDtype=Logical
  Out1 : Outport
  wires:
  Counter/1 -> Compare To Constant/1
  Constant/1 -> Counter/2
  Compare To Constant/1 -> Out1/1
  In1/1 -> Counter/1
